simulink model "Flying_capacitor_boost_simulink"  (R2021a)
settings: Solver=FixedStepDiscrete  StartTime=0.0  StopTime=2  FixedStep=sampleTime  MaxStep=1e-4  RelTol=1e-4  EnableMultiTasking=on
InitFcn:
  | flying_capacitor_parameters
model workspace (MAT data in the model file):
  Phase1 = 0
values from neighbouring files (symbols this model uses):
  Cfly = Cfly/2    (= 2.31481481481e-05)    [flying_capacitor_parameters.m]
  Cout = (IoutOneModule*D)/(SwitchingFrequency*DeltaVout)    [calculations.m]    (also in flying_capacitor_parameters.m = 2.31481481481e-05)
  D = (1-Vin/Vout)    (= 0.25)    [boost_parameters.m]    (also in calculations.m = (1-VinOneModule/VoutOneModule); flying_capacitor_parameters.m; unbalance_boost.m)
  Lboost = ((Vin-Vout/2)*D)/(DeltaIL*fsw)    (= 0.00084375)    [flying_capacitor_parameters.m]
  ModuleAPhase = 0    [boost_parameters.m]    (also in flying_capacitor_parameters.m = 90; unbalance_boost.m)
  ModuleBPhase = 180    [boost_parameters.m]    (also in flying_capacitor_parameters.m = 270; unbalance_boost.m = 90)
  ModuleCPhase = 90    [boost_parameters.m]    (also in flying_capacitor_parameters.m = 0)
  ModuleDPhase = 270    [boost_parameters.m]    (also in flying_capacitor_parameters.m = 180)
  Rcoil = 1e-3    (= 0.001)    [boost_parameters.m]    (also in unbalance_boost.m)
  Rload = Vout^2/P    (= 72)    [flying_capacitor_parameters.m]
  sampleTime = 5e-7    (= 5e-07)    [boost_parameters.m]    (also in flying_capacitor_parameters.m; unbalance_boost.m = 5e-08)
  Vin = 900    [boost_parameters.m]    (also in flying_capacitor_parameters.m; main.m = 880; unbalance_boost.m)
libraries: spsSeriesRLCBranchLib x9, simulink x8, spsVoltageMeasurementLib x5, spsDiodeLib x4, spsTriangleGeneratorLib x4, spsMosfetLib x4, spsCurrentMeasurementLib x3, spsVariableResistorLib x1, spsDCVoltageSourceLib x1, spspowerguiLib x1
settings Model: Creator=The MathWorks, Inc.  LastModifiedBy=enes_
settings SolverCC: AlgebraicLoopSolver=TrustRegion  SolverResetMethod=Robust
settings OptimizationCC: EfficientFloat2IntCast=on  LifeSpan=inf
settings DebuggingCC: ReadBeforeWriteMsg=DisableAll  WriteAfterWriteMsg=DisableAll  WriteAfterReadMsg=DisableAll  UniqueDataStoreMsg=error  StrictBusMsg=ErrorOnBusTreatedAsVector  SFUnexpectedBacktrackingDiag=warning  SFNoUnconditionalDefaultTransitionDiag=warning  SFExecutionAtInitializationDiag=none  SFMachineParentedDataDiag=warning  ArithmeticOperatorsInVariantConditions=warning
settings ModelReferenceCC: UpdateModelReferenceTargets=IfOutOfDate
settings SFSimCC: SFSimEcho=off  SimUseLocalCustomCode=off  CustomCodeUndefinedFunction=UseInterfaceOnly
settings RTWCC: RTWUseLocalCustomCode=off
settings CodeAppCC: StateflowObjectComments=on
settings GRTTargetCC: TargetLangStandard=C89/C90 (ANSI)
settings ConfigComp: CovMetricSettings=dw  CovSaveCumulativeToWorkspaceVar=on  CovSaveSingleToWorkspaceVar=on  CovExternalEMLEnable=off
settings SimscapeCC: SimscapeNormalizeSystem=off  SimscapeNominalValues={1, 'bar'; 1, 'cm^3/s'; 1, 'bar*kg/s'; 1, 'kJ/kg'; 1, 'kW'; }

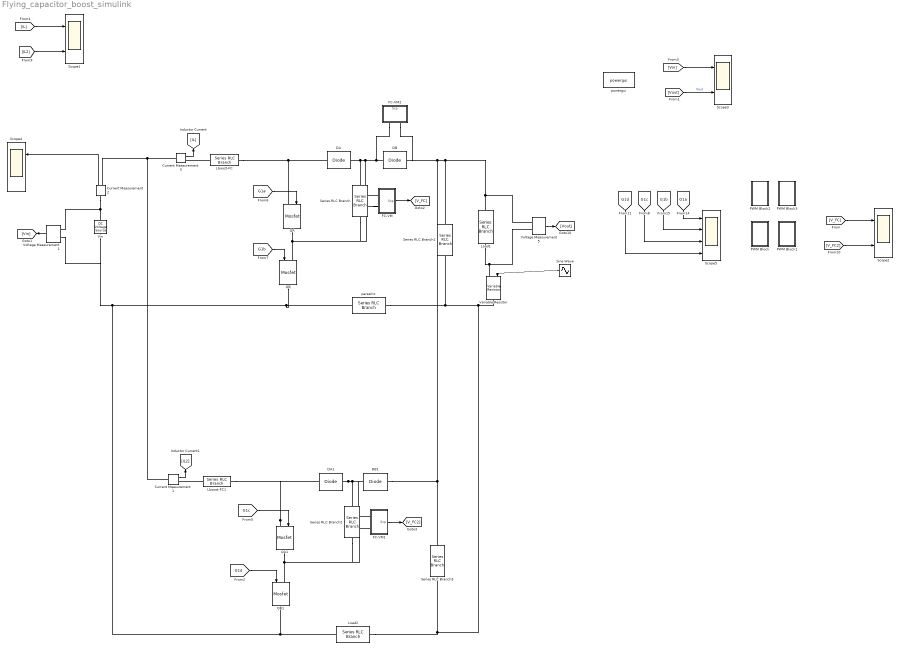
== system Flying_capacitor_boost_simulink ==
  Current Measurement1 : spsCurrentMeasurementLib/Current Measurement  PhasorSimulation=off  OutputType=Complex  PSBequivalent=0
  Current Measurement2 : spsCurrentMeasurementLib/Current Measurement  PhasorSimulation=off  OutputType=Complex  PSBequivalent=0
  Current Measurement3 : spsCurrentMeasurementLib/Current Measurement  PhasorSimulation=off  OutputType=Complex  PSBequivalent=0
  DA : spsDiodeLib/Diode  Ron=0.001  Lon=0  Vf=0.8  IC=0  UseSnubber=0  Rs=500  Cs=250e-9  Measurements=off
  DA1 : spsDiodeLib/Diode  Ron=0.001  Lon=0  Vf=0.8  IC=0  UseSnubber=0  Rs=500  Cs=250e-9  Measurements=off
  DB : spsDiodeLib/Diode  Ron=0.001  Lon=0  Vf=0.8  IC=0  UseSnubber=0  Rs=500  Cs=250e-9  Measurements=off
  DB1 : spsDiodeLib/Diode  Ron=0.001  Lon=0  Vf=0.8  IC=0  UseSnubber=0  Rs=500  Cs=250e-9  Measurements=off
  FC-VM : Subsystem
  FC-VM1 : Subsystem
  FC-VM2 : Subsystem
  Lboost-FC : spsSeriesRLCBranchLib/Series RLC Branch  LConnTagsString=__new0  RConnTagsString=__new0  BranchType=L  Resistance=Rcoil  Inductance=Lboost  SetiL0=off  InitialCurrent=11  Capacitance=1e-6  Setx0=off  InitialVoltage=0  Measurements=None
  Lboost-FC1 : spsSeriesRLCBranchLib/Series RLC Branch  LConnTagsString=__new0  RConnTagsString=__new0  BranchType=L  Resistance=Rcoil  Inductance=Lboost  SetiL0=off  InitialCurrent=11  Capacitance=1e-6  Setx0=off  InitialVoltage=0  Measurements=None
  Load1 : spsSeriesRLCBranchLib/Series RLC Branch  LConnTagsString=__new0  RConnTagsString=__new0  BranchType=R  Resistance=Rload  Inductance=200e-6  SetiL0=off  InitialCurrent=0  Capacitance=400e-6  Setx0=off  InitialVoltage=0  Measurements=None
  Load2 : spsSeriesRLCBranchLib/Series RLC Branch  LConnTagsString=__new0  RConnTagsString=__new0  BranchType=R  Resistance=Rload  Inductance=200e-6  SetiL0=off  InitialCurrent=0  Capacitance=400e-6  Setx0=off  InitialVoltage=0  Measurements=None
  PWM Block : Subsystem
  PWM Block1 : Subsystem
  PWM Block2 : Subsystem
  PWM Block3 : Subsystem
  QA : spsMosfetLib/Mosfet  Ron=0.1  Lon=0  Rd=0.01  Vfd=0  IC=0  Rs=1e5  Cs=inf  Measurements=off
  QA1 : spsMosfetLib/Mosfet  Ron=0.1  Lon=0  Rd=0.01  Vfd=0  IC=0  Rs=1e5  Cs=inf  Measurements=off
  QB : spsMosfetLib/Mosfet  Ron=0.1  Lon=0  Rd=0.01  Vfd=0  IC=0  Rs=1e5  Cs=inf  Measurements=off
  QB1 : spsMosfetLib/Mosfet  Ron=0.1  Lon=0  Rd=0.01  Vfd=0  IC=0  Rs=1e5  Cs=inf  Measurements=off
  Scope{1..4} (4 alike) : Scope  NumInputPorts=2
  Scope5 : Scope  NumInputPorts=4
  Series RLC Branch : spsSeriesRLCBranchLib/Series RLC Branch  LConnTagsString=__new0  RConnTagsString=__new0  BranchType=C  Resistance=1  Inductance=1e-3  SetiL0=off  InitialCurrent=0  Capacitance=Cfly  Setx0=off  InitialVoltage=600  Measurements=None
  Series RLC Branch1 : spsSeriesRLCBranchLib/Series RLC Branch  LConnTagsString=__new0  RConnTagsString=__new0  BranchType=C  Resistance=1  Inductance=1e-3  SetiL0=off  InitialCurrent=0  Capacitance=Cout  Setx0=off  InitialVoltage=1200  Measurements=None
  Series RLC Branch2 : spsSeriesRLCBranchLib/Series RLC Branch  LConnTagsString=__new0  RConnTagsString=__new0  BranchType=C  Resistance=1  Inductance=1e-3  SetiL0=off  InitialCurrent=0  Capacitance=Cfly  Setx0=off  InitialVoltage=600  Measurements=None
  Series RLC Branch3 : spsSeriesRLCBranchLib/Series RLC Branch  LConnTagsString=__new0  RConnTagsString=__new0  BranchType=C  Resistance=1  Inductance=1e-3  SetiL0=off  InitialCurrent=0  Capacitance=Cout  Setx0=off  InitialVoltage=1200  Measurements=None
  Sine Wave : Sin  Amplitude=0  Frequency=2*pi*150  SampleTime=0
  Variable Resistor : spsVariableResistorLib/Variable Resistor  Rabsmin=1e-3
      settings: SourceProductBaseCode=PS
  Vin : spsDCVoltageSourceLib/DC Voltage Source  Amplitude=Vin  Measurements=None
  Voltage Measurement1 : spsVoltageMeasurementLib/Voltage Measurement  PhasorSimulation=off  OutputType=Complex  PSBequivalent=0
  Voltage Measurement5 : spsVoltageMeasurementLib/Voltage Measurement  PhasorSimulation=off  OutputType=Complex  PSBequivalent=0
  parasitic : spsSeriesRLCBranchLib/Series RLC Branch  LConnTagsString=__new0  RConnTagsString=__new0  BranchType=R  Resistance=1e-4  Inductance=200e-6  SetiL0=off  InitialCurrent=0  Capacitance=400e-6  Setx0=off  InitialVoltage=0  Measurements=None
  powergui : spspowerguiLib/powergui  Priority=1  SimulationMode=Discrete  SampleTime=sampleTime  frequency=60  Iterations=50  frequencyindice=0  Pbase=100e6  ErrMax=1e-4  UnitsV=kV  UnitsW=MW  buscounter=0  FunctionMessages=off  echomessages=off  EnableUseOfTLC=off  CurrentSourceSwitches=off  DisableSnubberDevices=off  DisableRonSwitches=off  DisableVfSwitches=off  DisplayEquations=off  AutomaticDiscreteSolvers=off  SolverType=Tustin/Backward Euler (TBE)  Interpol=off  ExternalGateDelay=off  methode=off  Ts=100  x0status=blocks  SPID=on  SwTol=0  HookPort=off  NonlinearTolerance=1e-4  nMaxIteration=100  ContinueOnMaxIteration=off  RestoreLinks=warning  ResistiveCurrentMeasurement=off  Frange=[0:2:500]  Ylog=off  Xlog=on  ShowGrid=off  save=off  variable=ZData  structure=0  ZoomFFT=off  StartTime=0.0  cycles=1  DisplayStyle=1  fundamental=60  FreqAxis=off  MaxFrequency=1000  frequencyindicesteady=1  RmsSteady=1  display=off
  wires:
  Current Measurement3/1 -> [IL]
  Voltage Measurement5/1 -> [Vout]
  [G1a] -> QA/1
  [G1b] -> QB/1
  [G1a] -> Scope5/1
  [G1b] -> Scope5/2
  [Vout] -> Scope3/2  "Vout"
  Voltage Measurement1/1 -> [Vin]
  [Vin] -> Scope3/1
  [IL] -> Scope1/1
  FC-VM/1(Scp) -> [V_FC]
  [V_FC] -> Scope2/1
  [V_FC2] -> Scope2/2
  Sine Wave/1 -> Variable Resistor/1
  [G1d] -> QB1/1
  Current Measurement1/1 -> [IL2]
  FC-VM1/1(Scp) -> [V_FC2]
  [G1c] -> QA1/1
  [IL2] -> Scope1/2
  [G1c] -> Scope5/3
  [G1d] -> Scope5/4
  Current Measurement2/1 -> Scope4/1
  connections:
  Lboost-FC/LConn1 -- Current Measurement3/RConn1
  Voltage Measurement1/LConn1 -- Current Measurement2/LConn1 -- Vin/RConn1
  QA/RConn1 -- Series RLC Branch/RConn1 -- FC-VM/LConn2 -- QB/LConn1
  Lboost-FC/RConn1 -- DA/LConn1 -- QA/LConn1
  DB/LConn1 -- FC-VM2/LConn1 -- FC-VM/LConn1 -- Series RLC Branch/LConn1 -- DA/RConn1
  Load1/RConn1 -- Variable Resistor/LConn1 -- Voltage Measurement5/LConn2
  QA1/RConn1 -- Series RLC Branch2/RConn1 -- FC-VM1/LConn2 -- QB1/LConn1
  DA1/RConn1 -- Series RLC Branch2/LConn1 -- FC-VM1/LConn1 -- DB1/LConn1
  QA1/LConn1 -- DA1/LConn1 -- Lboost-FC1/RConn1
  Lboost-FC1/LConn1 -- Current Measurement1/RConn1
  DB1/RConn1 -- FC-VM2/LConn2 -- DB/RConn1 -- Series RLC Branch1/LConn1 -- Voltage Measurement5/LConn1 -- Load1/LConn1 -- Series RLC Branch3/LConn1
  Load2/RConn1 -- Vin/LConn1 -- Voltage Measurement1/LConn2 -- QB/RConn1 -- parasitic/RConn1 -- QB1/RConn1
  Load2/LConn1 -- Series RLC Branch1/RConn1 -- parasitic/LConn1 -- Variable Resistor/RConn1 -- Series RLC Branch3/RConn1
  Current Measurement1/LConn1 -- Current Measurement3/LConn1 -- Current Measurement2/RConn1

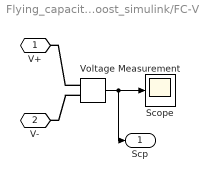
== system Flying_capacitor_boost_simulink/FC-VM ==
  Scope : Scope
  Voltage Measurement : spsVoltageMeasurementLib/Voltage Measurement  PhasorSimulation=off  OutputType=Complex  PSBequivalent=0
  V+ : PMIOPort  Side=Left
  V- : PMIOPort  Port=2  Side=Left
  Scp : Outport
  wires:
  Voltage Measurement/1 -> Scp/1, Scope/1
  connections:
  Voltage Measurement/LConn1 -- V+/RConn1
  Voltage Measurement/LConn2 -- V-/RConn1

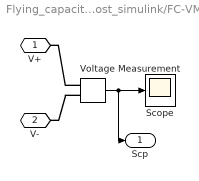
== system Flying_capacitor_boost_simulink/FC-VM1 ==
  Scope : Scope
  Voltage Measurement : spsVoltageMeasurementLib/Voltage Measurement  PhasorSimulation=off  OutputType=Complex  PSBequivalent=0
  V+ : PMIOPort  Side=Left
  V- : PMIOPort  Port=2  Side=Left
  Scp : Outport
  wires:
  Voltage Measurement/1 -> Scp/1, Scope/1
  connections:
  Voltage Measurement/LConn1 -- V+/RConn1
  Voltage Measurement/LConn2 -- V-/RConn1

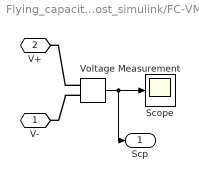
== system Flying_capacitor_boost_simulink/FC-VM2 ==
  Scope : Scope
  Voltage Measurement : spsVoltageMeasurementLib/Voltage Measurement  PhasorSimulation=off  OutputType=Complex  PSBequivalent=0
  V- : PMIOPort  Side=Left
  V+ : PMIOPort  Port=2  Side=Left
  Scp : Outport
  wires:
  Voltage Measurement/1 -> Scp/1, Scope/1
  connections:
  Voltage Measurement/LConn1 -- V+/RConn1
  Voltage Measurement/LConn2 -- V-/RConn1

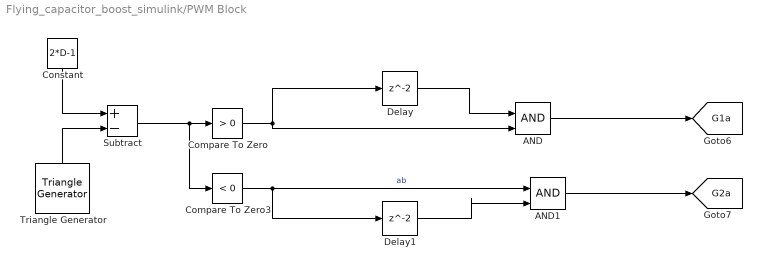
== system Flying_capacitor_boost_simulink/PWM Block ==
  AND : Logic  IconShape=distinctive  AllPortsSameDT=off  OutDataTypeStr=boolean
  AND1 : Logic  IconShape=distinctive  AllPortsSameDT=off  OutDataTypeStr=boolean
  Compare To Zero : simulink/Logic and Bit Operations/Compare To Zero  relop=>  OutDataTypeStr=boolean
  Compare To Zero3 : simulink/Logic and Bit Operations/Compare To Zero  relop=<  OutDataTypeStr=boolean
  Constant : Constant  Value=2*D-1
  Delay : Delay
  Delay1 : Delay
  Subtract : Sum  Inputs=+-
  Triangle Generator : spsTriangleGeneratorLib/Triangle Generator  Freq=fsw  Phase=ModuleAPhase  Ts=sampleTime
  tag scope: G1a=global, G2a=global
  wires:
  Constant/1 -> Subtract/1
  Triangle Generator/1 -> Subtract/2
  Subtract/1 -> Compare To Zero3/1, Compare To Zero/1
  AND/1 -> [G1a]
  Compare To Zero/1 -> Delay/1, AND/2
  Delay/1 -> AND/1
  Compare To Zero3/1 -> Delay1/1, AND1/1  "ab"
  AND1/1 -> [G2a]
  Delay1/1 -> AND1/2

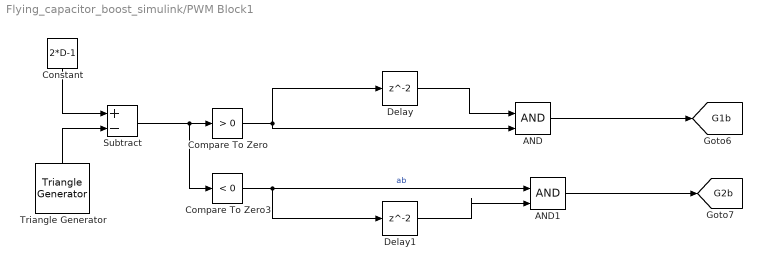
== system Flying_capacitor_boost_simulink/PWM Block1 ==
  AND : Logic  IconShape=distinctive  AllPortsSameDT=off  OutDataTypeStr=boolean
  AND1 : Logic  IconShape=distinctive  AllPortsSameDT=off  OutDataTypeStr=boolean
  Compare To Zero : simulink/Logic and Bit Operations/Compare To Zero  relop=>  OutDataTypeStr=boolean
  Compare To Zero3 : simulink/Logic and Bit Operations/Compare To Zero  relop=<  OutDataTypeStr=boolean
  Constant : Constant  Value=2*D-1
  Delay : Delay
  Delay1 : Delay
  Subtract : Sum  Inputs=+-
  Triangle Generator : spsTriangleGeneratorLib/Triangle Generator  Freq=fsw  Phase=ModuleBPhase  Ts=sampleTime
  tag scope: G1b=global, G2b=global
  wires:
  Constant/1 -> Subtract/1
  Triangle Generator/1 -> Subtract/2
  Subtract/1 -> Compare To Zero3/1, Compare To Zero/1
  AND/1 -> [G1b]
  Compare To Zero/1 -> Delay/1, AND/2
  Delay/1 -> AND/1
  Compare To Zero3/1 -> Delay1/1, AND1/1  "ab"
  AND1/1 -> [G2b]
  Delay1/1 -> AND1/2

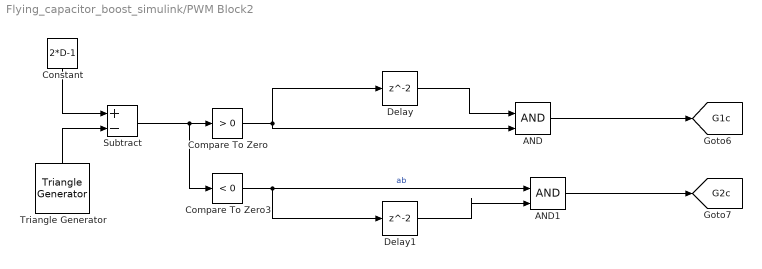
== system Flying_capacitor_boost_simulink/PWM Block2 ==
  AND : Logic  IconShape=distinctive  AllPortsSameDT=off  OutDataTypeStr=boolean
  AND1 : Logic  IconShape=distinctive  AllPortsSameDT=off  OutDataTypeStr=boolean
  Compare To Zero : simulink/Logic and Bit Operations/Compare To Zero  relop=>  OutDataTypeStr=boolean
  Compare To Zero3 : simulink/Logic and Bit Operations/Compare To Zero  relop=<  OutDataTypeStr=boolean
  Constant : Constant  Value=2*D-1
  Delay : Delay
  Delay1 : Delay
  Subtract : Sum  Inputs=+-
  Triangle Generator : spsTriangleGeneratorLib/Triangle Generator  Freq=fsw  Phase=ModuleCPhase  Ts=sampleTime
  tag scope: G1c=global, G2c=global
  wires:
  Constant/1 -> Subtract/1
  Triangle Generator/1 -> Subtract/2
  Subtract/1 -> Compare To Zero3/1, Compare To Zero/1
  AND/1 -> [G1c]
  Compare To Zero/1 -> Delay/1, AND/2
  Delay/1 -> AND/1
  Compare To Zero3/1 -> Delay1/1, AND1/1  "ab"
  AND1/1 -> [G2c]
  Delay1/1 -> AND1/2

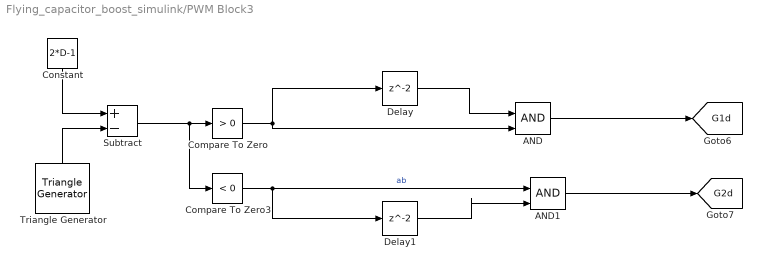
== system Flying_capacitor_boost_simulink/PWM Block3 ==
  AND : Logic  IconShape=distinctive  AllPortsSameDT=off  OutDataTypeStr=boolean
  AND1 : Logic  IconShape=distinctive  AllPortsSameDT=off  OutDataTypeStr=boolean
  Compare To Zero : simulink/Logic and Bit Operations/Compare To Zero  relop=>  OutDataTypeStr=boolean
  Compare To Zero3 : simulink/Logic and Bit Operations/Compare To Zero  relop=<  OutDataTypeStr=boolean
  Constant : Constant  Value=2*D-1
  Delay : Delay
  Delay1 : Delay
  Subtract : Sum  Inputs=+-
  Triangle Generator : spsTriangleGeneratorLib/Triangle Generator  Freq=fsw  Phase=ModuleDPhase  Ts=sampleTime
  tag scope: G1d=global, G2d=global
  wires:
  Constant/1 -> Subtract/1
  Triangle Generator/1 -> Subtract/2
  Subtract/1 -> Compare To Zero3/1, Compare To Zero/1
  AND/1 -> [G1d]
  Compare To Zero/1 -> Delay/1, AND/2
  Delay/1 -> AND/1
  Compare To Zero3/1 -> Delay1/1, AND1/1  "ab"
  AND1/1 -> [G2d]
  Delay1/1 -> AND1/2
